simulink model "Model"  (R2021a)
settings: Solver=ode4  StartTime=0.0  StopTime=inf  FixedStep=Ts  RelTol=1e-3
PreLoadFcn:
  | filepath  = fileparts(get_param(bdroot, 'FileName'))
  | cd(filepath);
values from neighbouring files (symbols this model uses):
  A_GRotation = [0 0 0]    [Parameter_PX4.m]
  ACC_UserFault = 0    [Parameter_PX4.m]
  ACCDrift = 0.0    (= 0)    [Parameter_PX4.m]
  ACCNoise = 1.0    (= 1)    [Parameter_PX4.m]
  accnoisegain = 0    [Parameter_PX4.m]
  ACCScale = 1.0    (= 1)    [Parameter_PX4.m]
  BaroNoise = 1.0    (= 1)    [Parameter_PX4.m]
  GyroDrift = 0.0    (= 0)    [Parameter_PX4.m]
  GyroNoise = 1.0    (= 1)    [Parameter_PX4.m]
  GyroScale = 1.0    (= 1)    [Parameter_PX4.m]
  MagDrift = 0.0    (= 0)    [Parameter_PX4.m]
  MagNoise = 1.0    (= 1)    [Parameter_PX4.m]
  MagRotation = [0 0 0]    [Parameter_PX4.m]
  MagScale = 1.0    (= 1)    [Parameter_PX4.m]
  ModelInit_GroundSlope = [0,0]    [Parameter_PX4.m]
  ModelInit_RPM = 0    [Parameter_PX4.m]
  ModelParam_envAltitude = -100    [Parameter_PX4.m]
  ModelParam_GlobalNoiseGainSwitch = 0.4    [Parameter_PX4.m]
  ModelParam_GPSEphFinal = 0.3    [Parameter_PX4.m]
  ModelParam_GPSEpvFinal = 0.4    [Parameter_PX4.m]
  ModelParam_GPSFix3DFix = 3    [Parameter_PX4.m]
  ModelParam_GPSSatsVisible = 10    [Parameter_PX4.m]
  ModelParam_motorCr = 842.1    [Parameter_PX4.m]
  ModelParam_motorJm = 0.0001287    [Parameter_PX4.m]
  ModelParam_motorMinThr = 0.05    [Parameter_PX4.m]
  ModelParam_motorT = 0.0214    [Parameter_PX4.m]
  ModelParam_motorWb = 22.83    [Parameter_PX4.m]
  ModelParam_noiseBaroCoupleWithSpeed = 0    [Parameter_PX4.m]
  ModelParam_noiseUpperWindBodyRatio = 0    [Parameter_PX4.m]
  ModelParam_rotorCm = 2.783e-07    [Parameter_PX4.m]
  ModelParam_rotorCt = 1.681e-05    [Parameter_PX4.m]
  ModelParam_uavCCm = [0.0035 0.0039 0.0034]    [Parameter_PX4.m]
  ModelParam_uavCd = 0.055    [Parameter_PX4.m]
  ModelParam_uavDearo = 0.12    [Parameter_PX4.m]
  ModelParam_uavMass = 1.515    [Parameter_PX4.m]
  ModelParam_uavR = 0.225    [Parameter_PX4.m]
  ModelParam_uavType = int8(3)    [Parameter_PX4.m]
  MyNoiseGain = [2.5;3;4].*3    [Parameter_PX4.m]
  PWMNoiseGain = [10;15;3]    [Parameter_PX4.m]
  TemperatureConstant = 25.0    (= 25)    [Parameter_PX4.m]
  Ts = 1/2000    (= 0.0005)    [Parameter_PX4.m]
  TypeMotorAngMatrix = [     [pi/3 pi -pi/3 0 0 0 0 0];     [pi/3 pi -pi/3 0 0 0 0 0];     [pi/4 pi/4+pi pi/4+3*pi/2 pi/4+pi/2 0 0 0 0];     [pi/2 3*pi/2 0 pi 0 0 0 0];     [pi/2 3/2*pi 3/2*pi+pi/3 pi/2+pi/3 pi/2-pi/3 3/2*pi-pi/3 0 0];     [0 pi pi+pi/3 pi/3 -pi/3 pi-pi/3 0 0];     [pi/3 pi/3 pi pi -pi/3 -pi/3 0 0];     [pi/8 pi+pi/8 pi/8+pi/4 pi-pi/8 -pi/8 3/2*pi-pi/8 3/2*pi+pi/8 pi/2+pi/8];     [0 pi pi/4 3/4*pi -pi/4 ...(+86 chars)    [Parameter_PX4.m]
  TypeMotorDirMatrix = [     [-1 -1 -1 0 0 0 0 0];     [1 1 1 0 0 0 0 0];     [-1 -1 1 1 0 0 0 0];     [-1 -1 1 1 0 0 0 0];     [1 -1 1 -1 -1 1 0 0];     [1 -1 1 -1 -1 1 0 0];     [1 -1 1 -1 1 -1 0 0];     [1 1 -1 -1 -1 -1 1 1];     [1 1 -1 -1 -1 -1 1 1];     [-1 1 -1 1 -1 1 -1 1]; ]'    [Parameter_PX4.m]
  TypeMotorNonVector = int8([3;3;4;4;6;6;6;8;8;8])    [Parameter_PX4.m]
undefined symbols (not defined in the file or in its folder): Earth, ModelParam_GPSEpvInitial, ModelParam_GPSEpvTimeConstant, ModelParam_noiseGPSSampTime, ModelParam_noisePowerIMU, ModelParam_noisePowerOffGainAccel, ModelParam_noisePowerOffGainAccelZ, ModelParam_noisePowerOffGainGyro, ModelParam_noisePowerOffGainGyroZ, ModelParam_noisePowerOffGainMag, ModelParam_noisePowerOffGainMagZ, ModelParam_noisePowerOnGainAccel, ModelParam_noisePowerOnGainAccelZ, ModelParam_noisePowerOnGainGyro, ModelParam_noisePowerOnGainGyroZ, ModelParam_noisePowerOnGainMag, ModelParam_noisePowerOnGainMagZ, ModelParam_noiseUpperGPS, ModelParam_timeSamp, Newton, Raphson, WGS84
libraries: simulink x11, sharedtransform x7, aerolibutil x4, aerolibtransform2 x4, aerolibasang x3, simulink_extras x2, etargetslib x2, aerolibatmos2 x2, shared6dof x1, aerolibconvert2 x1, aerolibobsolete x1, aerolibnav x1
(part 1 of 3)
settings Model: SimulationMode=accelerator  ParamWorkspaceSource=ReferencedWorkspace  Creator=Jinrui  LastModifiedBy=fangr
settings SolverCC: AlgebraicLoopSolver=TrustRegion  PositivePriorityOrder=on  AutoInsertRateTranBlk=on
settings DataIOCC: ReturnWorkspaceOutputs=off
settings OptimizationCC: BlockReduction=off  EnhancedBackFolding=on  PassReuseOutputArgsAs=Individual arguments  ZeroExternalMemoryAtStartup=off  ZeroInternalMemoryAtStartup=off  OptimizeBlockOrder=speed  DifferentSizesBufferReuse=on  OptimizationCustomize=off  EfficientTunableParamExpr=on
settings DebuggingCC: ParameterTunabilityLossMsg=error  SFMachineParentedDataDiag=warning  ArithmeticOperatorsInVariantConditions=warning
settings HardwareCC: ProdBitPerPointer=32  ProdBitPerSizeT=32  ProdBitPerPtrDiffT=32  ProdLargestAtomicInteger=Long  ProdLargestAtomicFloat=Double  ProdWordSize=32  ProdHWDeviceType=ARM Compatible->ARM Cortex-A
settings SFSimCC: SimUseLocalCustomCode=off  MATLABDynamicMemAlloc=off  CustomCodeUndefinedFunction=UseInterfaceOnly
settings RTWCC: SystemTargetFile=ert.tlc  GenCodeOnly=on  PackageGeneratedCodeAndArtifacts=on  PackageName=Model  TemplateMakefile=ert_default_tmf  GenerateReport=on  RTWUseLocalCustomCode=off  Toolchain=Linaro Toolchain v4.8  BuildConfiguration=Faster Runs  DLArmComputeVersion=20.02.1
settings CodeAppCC: IgnoreCustomStorageClasses=off  OperatorAnnotations=on  SimulinkDataObjDesc=on  SFDataObjDesc=on  SimulinkBlockComments=off
settings ERTTargetCC: TargetLangStandard=C99 (ISO)  GenerateSampleERTMain=on  SupportComplex=off  SupportContinuousTime=on  SupportVariableSizeSignals=on  RootIOFormat=Structure reference  ERTCustomFileTemplate=example_file_process.tlc  ERTFilePackagingFormat=Compact
settings SimscapeCC: SimscapeNormalizeSystem=off
settings ConfigComp: DVTestSuiteOptimization=Auto  DVDetectOutOfBounds=on  DVModelReferenceHarness=on  DVHarnessSource=Signal Editor

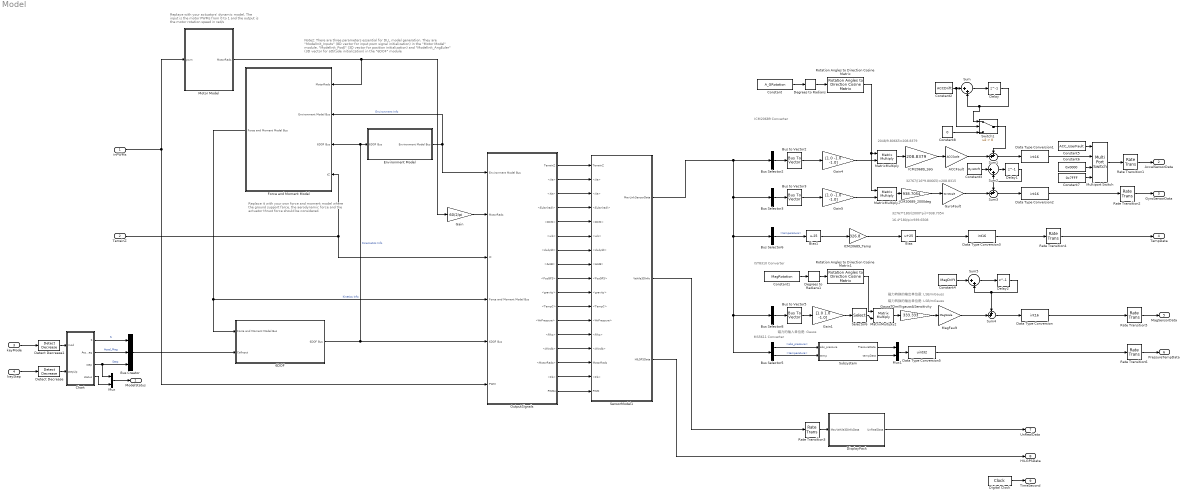
== system Model ==
  note: Replace it with your own force and moment model
      | where the ground support farce, the aerodynamic force
      | and the actuator thrust force should be considered.
  note: Replace with your actuators' dynamic model,
      | The input is the motor PWMs from 0 to 1
      | and the output is the motor rotation speed in rad/s
  note: Note2: There are three parameters essential for DLL model generation. They are "ModelInit_Inputs" (8D vector for input pwm signal initialization) in the "Motor Model" module, "ModelInit_PosE" (3D vector for position initialization) and "ModelInit_AngEuler" (3D vector for attitude initialization) in the "6DOF" module
  note: ICM20689 Converter
  note: 32767/(16*9.80665)=208.8315
  note: 2048/9.80665=208.8379
  note: 32767*180/(2000*pi)=938.7054
  note: IST8310 Converter
  note: 磁力转换的输出单位是: LSB/mGauss
  note: 磁力的输入单位是: Gauss
  note: MS5611 Converter
  note: 16.4*180/pi=939.6508
  note: 磁力转换的输出单位是: LSB/mGauss
  inPWMs : Inport  PortDimensions=8
  TerrainZ : Inport  Port=2  SampleTime=1
  keyMode : Inport  Port=3
  keyStep : Inport  Port=4
  6DOF : Subsystem
  ACCFault : Gain  Gain=ACCScale  OutDataTypeStr=double  RndMeth=Nearest
  Bias : Bias  Bias=25
  Bias1 : Bias  Bias=-25
  Bus Creator : BusCreator  Inputs=3
  Bus Selector2 : BusSelector  OutputSignals=xacc,yacc,zacc  OutputAsBus=on
  Bus Selector3 : BusSelector  OutputSignals=xgyro,ygyro,zgyro  OutputAsBus=on
  Bus Selector5 : BusSelector  OutputSignals=abs_pressure,temperature
  Bus Selector6 : BusSelector  OutputSignals=temperature
  Bus Selector8 : BusSelector  OutputSignals=xmag,ymag,zmag  OutputAsBus=on
  Bus to Vector2 : BusToVector
  Bus to Vector3 : BusToVector
  Bus to Vector5 : BusToVector
  Chart : Stateflow chart  TreatAsAtomicUnit=on
  Constant : Constant  Value=A_GRotation
  Constant1 : Constant  Value=MagRotation
  Constant2 : Constant  Value=ACCDrift
  Constant3 : Constant  Value=GyroDrift
  Constant4 : Constant  Value=MagDrift
  Constant5 : Constant  Value=ACC_UserFault
  Constant6 : Constant  Value=0x0000  OutDataTypeStr=int16
  Constant7 : Constant  Value=0x7FFF  OutDataTypeStr=int16
  Constant8 : Constant  Value=0
  Data Type Conversion : DataTypeConversion  OutDataTypeStr=int16  RndMeth=Nearest
  Data Type Conversion1 : DataTypeConversion  OutDataTypeStr=int16  RndMeth=Nearest  SaturateOnIntegerOverflow=on
  Data Type Conversion2 : DataTypeConversion  OutDataTypeStr=int16  RndMeth=Nearest  SaturateOnIntegerOverflow=on
  Data Type Conversion3 : DataTypeConversion  OutDataTypeStr=int16  RndMeth=Nearest
  Data Type Conversion5 : DataTypeConversion  OutDataTypeStr=uint32  RndMeth=Nearest
  Degrees to Radians : simulink_extras/Transformations/Degrees to Radians
  Degrees to Radians1 : simulink_extras/Transformations/Degrees to Radians
  Delay : Delay  DelayLength=1
  Delay1 : Delay  DelayLength=1
  Delay2 : Delay  DelayLength=1
  Detect Decrease : simulink/Logic and Bit Operations/Detect Decrease  vinit=0.0  OutDataTypeStr=boolean
  Detect Decrease1 : simulink/Logic and Bit Operations/Detect Decrease  vinit=0.0  OutDataTypeStr=boolean
  Digital Clock : DigitalClock  SampleTime=Ts
  DisplayPack : Subsystem  TreatAsAtomicUnit=on  SystemSampleTime=Ts
  Environment Model : Subsystem
  Force and Moment Model : Subsystem
  Gain : Gain  Gain=60/2/pi
  Gain1 : Gain  Gain=[1.0 1.0 -1.0]  RndMeth=Nearest
  Gain4 : Gain  Gain=[1.0 -1.0 -1.0]  RndMeth=Nearest
  Gain5 : Gain  Gain=[1.0 -1.0 -1.0]  RndMeth=Nearest
  GaussTOmilligauss&Sensitivity : Gain  Gain=333.333  OutDataTypeStr=double  RndMeth=Nearest
  GyroFault : Gain  Gain=GyroScale  OutDataTypeStr=double  RndMeth=Nearest
  ICM20689_16G : Gain  Gain=208.8379  OutDataTypeStr=double  RndMeth=Nearest
  ICM20689_2000deg : Gain  Gain=938.7054  OutDataTypeStr=double  RndMeth=Nearest
  ICM20689_Temp : Gain  Gain=326.8  OutDataTypeStr=double
  MagFault : Gain  Gain=MagScale  OutDataTypeStr=double  RndMeth=Nearest
  MatrixMultiply : Product  Multiplication=Matrix(*)
  MatrixMultiply1 : Product  Multiplication=Matrix(*)
  MatrixMultiply2 : Product  Multiplication=Matrix(*)
  Motor Model : Subsystem
  Multiport Switch : MultiPortSwitch  DataPortOrder=Specify indices  DataPortIndices={0,1,2}  DiagnosticForDefault=None
  Mux : Mux  Inputs=2
  Mux1 : Mux  Inputs=2
  OutputSignals : Subsystem
  Rate Transition1 : RateTransition  OutPortSampleTime=Ts*2
  Rate Transition2 : RateTransition  OutPortSampleTime=Ts
  Rate Transition3 : RateTransition  OutPortSampleTime=0.01
  Rate Transition4 : RateTransition  OutPortSampleTime=Ts
  Rate Transition5 : RateTransition  OutPortSampleTime=Ts
  Rate Transition6 : RateTransition  OutPortSampleTime=Ts*2
  Rotation Angles to Direction Cosine Matrix : sharedtransform/Rotation Angles to Direction Cosine Matrix  rotationOrder=ZYX  aMode=aMode
      settings: SourceProductBaseCode=AE,PW,DR,MT,VE
  Rotation Angles to Direction Cosine Matrix1 : sharedtransform/Rotation Angles to Direction Cosine Matrix  rotationOrder=ZYX  aMode=aMode
      settings: SourceProductBaseCode=AE,PW,DR,MT,VE
  Selector6 : Selector  InputPortWidth=3  IndexOptions=Index vector (dialog)  Indices=[2 1 3]  OutputSizes=1
  SensorModel1 : Subsystem
  Subsystem : Subsystem
  Sum : Sum  Inputs=|++
  Sum1 : Sum  Inputs=++|
  Sum2 : Sum  Inputs=|++
  Sum3 : Sum  Inputs=++|
  Sum4 : Sum  Inputs=++|
  Sum5 : Sum  Inputs=|++
  Switch1 : Switch  Criteria=u2 > Threshold
  ModelStatus : Outport  PortDimensions=2
  AccelSensorData : Outport  Port=2  OutDataTypeStr=int16
  GyroSensorData : Outport  Port=3
  TempData : Outport  Port=4
  MagSensorData : Outport  Port=5
  PressureTempData : Outport  Port=6
  UnRealData : Outport  Port=7
  HILGPSData : Outport  Port=8
  TimeSecond : Outport  Port=9
  wires:
  inPWMs/1 -> Motor Model/1(pwm), OutputSignals/6(PWM)
  OutputSignals/7(<dwb/dt>) -> SensorModel1/7(<dwb/dt>)
  OutputSignals/13(<Rho>) -> SensorModel1/13(<Rho>)
  OutputSignals/6(<wb>) -> SensorModel1/6(<wb>)
  OutputSignals/12(<AirPressure>) -> SensorModel1/12(<AirPressure>)
  OutputSignals/9(<PosGPS>) -> SensorModel1/9(<PosGPS>)
  Environment Model/1(Environment Model Bus) -> Force and Moment Model/2(Environment Model Bus), OutputSignals/1(Environment Model Bus)  "Environment Info"
  OutputSignals/17(PWMs) -> SensorModel1/17(PWM)
  OutputSignals/11(<TempC>) -> SensorModel1/11(<TempC>)
  OutputSignals/10(<gravity>) -> SensorModel1/10(<gravity>)
  TerrainZ/1 -> Force and Moment Model/4("tZ "), OutputSignals/3(zt)
  OutputSignals/8(<AccB>) -> SensorModel1/8(<AccB>)
  Chart/3(step) -> Mux/1, Bus Creator/3  "Step"
  Chart/2(Accel_Mag) -> Bus Creator/2  "Accel_Mag"
  Detect Decrease1/1 -> Chart/1(mod)
  Force and Moment Model/1(Force and Moment Model Bus) -> OutputSignals/4(Force and Moment Model Bus), 6DOF/1(Force and Moment Model Bus)  "Kinetics Info"
  OutputSignals/2(<Ve>) -> SensorModel1/2(<Ve>)
  OutputSignals/1(TerrainZ) -> SensorModel1/1(TerrainZ)
  OutputSignals/4(<Eular(rad)>) -> SensorModel1/4(<Eular(rad)>)
  6DOF/1(6DOF Bus) -> Force and Moment Model/3(6DOF Bus), Environment Model/1(6DOF Bus), OutputSignals/5(6DOF Bus)  "Kinematics Info"
  OutputSignals/3(<Xe>) -> SensorModel1/3(<Xe>)
  Motor Model/1(MotorRads) -> Force and Moment Model/1(MotorRads), Gain/1
  OutputSignals/15(<MotorRads>) -> SensorModel1/15(MotorRads)
  OutputSignals/16(<Fb>) -> SensorModel1/16(<Fb>)
  OutputSignals/14(<Windb>) -> SensorModel1/14(<Windb>)
  Detect Decrease/1 -> Chart/2(stepUp)
  keyMode/1 -> Detect Decrease1/1
  Chart/4(status) -> Mux/2
  Chart/1(S) -> Bus Creator/1  "S"
  OutputSignals/5(<DCM>) -> SensorModel1/5(<DCM>)
  keyStep/1 -> Detect Decrease/1
  Bus Creator/1 -> 6DOF/2(CalInput)
  Mux/1 -> ModelStatus/1
  Gain/1 -> OutputSignals/2(MotorRads)
  Sum2/1 -> Delay1/1
  ACCFault/1 -> Sum1/2
  Constant3/1 -> Sum2/1
  Delay1/1 -> Sum3/1, Sum2/2
  ICM20689_Temp/1 -> Bias/1
  Delay/1 -> Switch1/1, Sum/2
  Degrees to Radians1/1 -> Rotation Angles to Direction Cosine Matrix1/1
  Bus Selector5/1 -> Subsystem/1(abs_pressure)  "<abs_pressure>"
  Rotation Angles to Direction Cosine Matrix1/1 -> MatrixMultiply2/1
  MagFault/1 -> Sum4/2
  GyroFault/1 -> Sum3/2
  Sum/1 -> Delay/1
  SensorModel1/2(Vehile3DInfo) -> Rate Transition3/1
  Constant1/1 -> Degrees to Radians1/1
  MatrixMultiply1/1 -> ICM20689_2000deg/1
  Subsystem/2(tempData) -> Mux1/2
  Constant4/1 -> Sum5/1
  Rate Transition3/1 -> DisplayPack/1(MavVehile3DInfoData)
  Sum5/1 -> Delay2/1
  Sum3/1 -> Data Type Conversion2/1
  ICM20689_16G/1 -> ACCFault/1
  ICM20689_2000deg/1 -> GyroFault/1
  Bus Selector8/1 -> Bus to Vector5/1
  SensorModel1/1(MavLinkSensorData) -> Bus Selector3/1, Bus Selector6/1, Bus Selector8/1, Bus Selector5/1, Bus Selector2/1
  DisplayPack/1(UnRealData) -> UnRealData/1
  Mux1/1 -> Data Type Conversion5/1
  Sum4/1 -> Data Type Conversion/1
  Delay2/1 -> Sum4/1, Sum5/2
  Selector6/1 -> MatrixMultiply2/2
  Bus Selector6/1 -> Bias1/1  "<temperature>"
  Bias/1 -> Data Type Conversion3/1
  Sum1/1 -> Data Type Conversion1/1
  Bus Selector3/1 -> Bus to Vector3/1
  Degrees to Radians/1 -> Rotation Angles to Direction Cosine Matrix/1
  Constant2/1 -> Switch1/2, Sum/1
  Bus Selector2/1 -> Bus to Vector2/1
  Bus to Vector5/1 -> Gain1/1
  Bias1/1 -> ICM20689_Temp/1
  Bus to Vector3/1 -> Gain5/1
  SensorModel1/3(HILGPSData) -> HILGPSData/1
  Gain1/1 -> Selector6/1
  Constant/1 -> Degrees to Radians/1
  Subsystem/1(PressureData) -> Mux1/1
  Bus Selector5/2 -> Subsystem/2(temp)  "<temperature>"
  MatrixMultiply2/1 -> GaussTOmilligauss&Sensitivity/1
  Gain4/1 -> MatrixMultiply/2
  GaussTOmilligauss&Sensitivity/1 -> MagFault/1
  MatrixMultiply/1 -> ICM20689_16G/1
  Bus to Vector2/1 -> Gain4/1
  Constant5/1 -> Multiport Switch/1
  Data Type Conversion1/1 -> Multiport Switch/2
  Constant6/1 -> Multiport Switch/3
  Constant7/1 -> Multiport Switch/4
  Gain5/1 -> MatrixMultiply1/2
  Digital Clock/1 -> TimeSecond/1
  Multiport Switch/1 -> Rate Transition1/1
  Rate Transition1/1 -> AccelSensorData/1
  Rate Transition2/1 -> GyroSensorData/1
  Data Type Conversion2/1 -> Rate Transition2/1
  Rate Transition4/1 -> TempData/1
  Data Type Conversion3/1 -> Rate Transition4/1
  Data Type Conversion/1 -> Rate Transition5/1
  Rate Transition5/1 -> MagSensorData/1
  Data Type Conversion5/1 -> Rate Transition6/1
  Rate Transition6/1 -> PressureTempData/1
  Rotation Angles to Direction Cosine Matrix/1 -> MatrixMultiply/1, MatrixMultiply1/1
  Constant8/1 -> Switch1/3
  Switch1/1 -> Sum1/1

== system Model/6DOF ==
  Force and Moment Model Bus : Inport
  CalInput : Inport  Port=2
  Bus Creator : BusCreator  Inputs=8
  Bus Selector : BusSelector  OutputSignals=Step,Accel_Mag,S
  Bus Selector1 : BusSelector  OutputSignals=Fb,Mb
  CaliModel : Subsystem
  Custom Variable Mass 6DOF (Quaternion) : shared6dof/6DOF (Euler Angles)  units=Metric (MKS)  mtype=Fixed  rep=Quaternion  xme_0=ModelInit_PosE  Vm_0=ModelInit_VelB  eul_0=ModelInit_AngEuler  pm_0=ModelInit_RateB  mass_0=ModelParam_uavMass  mass_e=0.5  mass_f=2.0  inertia=ModelParam_uavJ  inertia_e=eye(3)  inertia_f=2*eye(3)  k_quat=1.0  vre_flag=off  abi_flag=off  aMode=aMode  xme_statename=''  Vm_statename=''  eul_statename=''  quat_statename=''  pm_statename=''  mass_statename=''
      settings: SourceProductBaseCode=AE,PW,DR,MT,VE
  Demux2 : Demux  Outputs=3
  Mux : Mux  Inputs=3
  Switch : Switch  Criteria=u2 > Threshold
  Switch1 : Switch  Criteria=u2 > Threshold
  Wrap To Zero : simulink/Discontinuities/Wrap To Zero  Threshold=0
      settings: SourceProductBaseCode=SL
  6DOF Bus : Outport  VectorParamsAs1DForOutWhenUnconnected=off
  wires:
  Bus Selector1/1 -> Switch/1  "<Fb>"
  Custom Variable Mass 6DOF (Quaternion)/8 -> Bus Creator/8  "AccB"
  Custom Variable Mass 6DOF (Quaternion)/5 -> Bus Creator/5  "Vb"
  Custom Variable Mass 6DOF (Quaternion)/6 -> Bus Creator/6, CaliModel/3(wb)  "wb"
  Custom Variable Mass 6DOF (Quaternion)/1 -> Bus Creator/1  "Ve"
  Custom Variable Mass 6DOF (Quaternion)/4 -> CaliModel/4(DCM_be), Bus Creator/4  "DCM"
  Custom Variable Mass 6DOF (Quaternion)/3 -> Bus Creator/3  "Eular(rad)"
  Custom Variable Mass 6DOF (Quaternion)/7 -> Bus Creator/7  "dwb/dt"
  Bus Selector1/2 -> Switch1/1  "<Mb>"
  Force and Moment Model Bus/1 -> Bus Selector1/1
  Bus Creator/1 -> 6DOF Bus/1
  Bus Selector/3 -> Switch/2, Switch1/2  "<S>"
  Bus Selector/2 -> CaliModel/2(Accel_Mag)  "<Accel_Mag>"
  Bus Selector/1 -> CaliModel/1(step)  "<Step>"
  CalInput/1 -> Bus Selector/1
  Switch/1 -> Custom Variable Mass 6DOF (Quaternion)/1
  Switch1/1 -> Custom Variable Mass 6DOF (Quaternion)/2
  CaliModel/1(Fb) -> Switch/3
  CaliModel/2(Mb) -> Switch1/3
  Demux2/1 -> Mux/1
  Demux2/2 -> Mux/2
  Demux2/3 -> Wrap To Zero/1
  Wrap To Zero/1 -> Mux/3
  Custom Variable Mass 6DOF (Quaternion)/2 -> Demux2/1  "Xe"
  Mux/1 -> Bus Creator/2  "Xe"

== system Model/DisplayPack ==
  MavVehile3DInfoData : Inport
  Bus Selector : BusSelector  OutputSignals=copterID,vehicleType,runnedTime,VelE,PosE,AngEuler,AngQuatern,MotorRPMS,AccB,RateB,PosGPS
  UnRealDataPackege : Subsystem  TreatAsAtomicUnit=on
  UnRealData : Outport
  wires:
  UnRealDataPackege/1(toUnReal) -> UnRealData/1
  MavVehile3DInfoData/1 -> Bus Selector/1
  Bus Selector/1 -> UnRealDataPackege/1(copterID)  "<copterID>"
  Bus Selector/2 -> UnRealDataPackege/2(vehicleType)  "<vehicleType>"
  Bus Selector/3 -> UnRealDataPackege/3(runnedTime)  "<runnedTime>"
  Bus Selector/4 -> UnRealDataPackege/4("VelE ")  "<VelE>"
  Bus Selector/5 -> UnRealDataPackege/5(PosE)  "<PosE>"
  Bus Selector/6 -> UnRealDataPackege/6(AngEuler)  "<AngEuler>"
  Bus Selector/7 -> UnRealDataPackege/7(AngQuatern)  "<AngQuatern>"
  Bus Selector/8 -> UnRealDataPackege/8(MotorRPMS)  "<MotorRPMS>"
  Bus Selector/9 -> UnRealDataPackege/9(AccB)  "<AccB>"
  Bus Selector/10 -> UnRealDataPackege/10(RateB)  "<RateB>"
  Bus Selector/11 -> UnRealDataPackege/11(PosGPS)  "<PosGPS>"

== system Model/Environment Model ==
  6DOF Bus : Inport
  Bus Creator : BusCreator  Inputs=6
  Bus Selector : BusSelector  OutputSignals=Xe,Vb
  Constant_[1 1 1] : Constant  Value=[1,1,1]  VectorParams1D=off
  Flat Earth to LLA : aerolibtransform2/Flat Earth to LLA  units=Metric (MKS)  ptype=Earth (WGS84)  F=1/298.257223563  R=6378137  refPosPort=off  LL0=ModelParam_GPSLatLong  psi=0
  ISA Atmosphere Model : aerolibatmos2/ISA Atmosphere Model  custom=off  g=9.80665  gamma=1.4  R=287.0531  L=0.0065  h_trop=11000  h_strat=20000  rho0=1.225  P0=101325  T0=288.15  h0=0
  ModelParam.envAltitude : Constant  Value=ModelParam_envAltitude
  ModelParam.noiseUpperWindBodyRatio : Gain  Gain=ModelParam_noiseUpperWindBodyRatio
  ModelParam.noiseUpperWindBodyRatioSwitch : Gain  Gain=ModelParam_GlobalNoiseGainSwitch
  Mux : Mux  Inputs=2
  Product1 : Product
  Reshape : Reshape
  Saturation : Saturate  UpperLimit=100000  LowerLimit=0
  Sum1 : Sum  Inputs=|++
  Temperature Conversion : aerolibconvert2/Temperature Conversion  IU=K  OU=C
      settings: SourceProductBaseCode=AE
  TemperatureConstant : Constant  Value=TemperatureConstant
  Terminator2 : Terminator
  Terminator3 : Terminator
  Uniform Random Number : UniformRandomNumber  Minimum=[-1,-1,-0.5]  Maximum=[1,1,0.5]  Seed=[564565,6846798,46545]  SampleTime=Ts
  "WGS84 Gravity Model " : aerolibobsolete/WGS84 Gravity Model   model=WGS84 Taylor Series  units=Metric (MKS)  no_atmos=on  precessing=on  jd_loc=off  month=October  day=10  year=2004  no_centrifugal=on  action=Warning
      settings: SourceProductBaseCode=AE
  Environment Model Bus : Outport  VectorParamsAs1DForOutWhenUnconnected=off
  wires:
  ModelParam.envAltitude/1 -> Flat Earth to LLA/2
  Bus Creator/1 -> Environment Model Bus/1
  Bus Selector/1 -> Flat Earth to LLA/1  "<Xe>"
  Constant_[1 1 1]/1 -> Sum1/1
  ModelParam.noiseUpperWindBodyRatioSwitch/1 -> Sum1/2
  ModelParam.noiseUpperWindBodyRatio/1 -> ModelParam.noiseUpperWindBodyRatioSwitch/1
  6DOF Bus/1 -> Bus Selector/1
  ISA Atmosphere Model/3 -> Bus Creator/4  "AirPressure"
  "WGS84 Gravity Model "/1 -> Reshape/1
  TemperatureConstant/1 -> Bus Creator/3  "TempC"
  ISA Atmosphere Model/4 -> Bus Creator/5  "Rho"
  Uniform Random Number/1 -> ModelParam.noiseUpperWindBodyRatio/1
  Reshape/1 -> Bus Creator/2  "gravity"
  Product1/1 -> Bus Creator/6  "Windb"
  Flat Earth to LLA/1 -> Mux/1
  Temperature Conversion/1 -> Terminator2/1
  Mux/1 -> Bus Creator/1, "WGS84 Gravity Model "/1  "PosGPS"
  ISA Atmosphere Model/2 -> Terminator3/1
  ISA Atmosphere Model/1 -> Temperature Conversion/1
  Bus Selector/2 -> Product1/2  "<Vb>"
  Flat Earth to LLA/2 -> Mux/2, Saturation/1
  Sum1/1 -> Product1/1
  Saturation/1 -> ISA Atmosphere Model/1

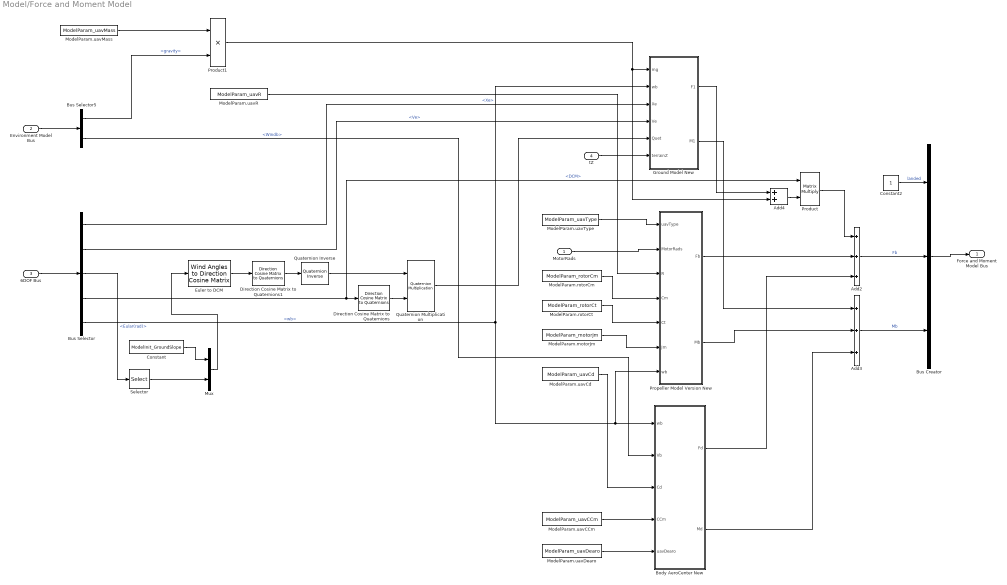
== system Model/Force and Moment Model ==
  MotorRads : Inport
  Environment Model Bus : Inport  Port=2
  6DOF Bus : Inport  Port=3
  "tZ " : Inport  Port=4
  Add2 : Sum  Inputs=+++
  Add3 : Sum  Inputs=+++
  Add4 : Sum
  Body AeroCenter New : Subsystem
  Bus Creator : BusCreator  Inputs=3
  Bus Selector : BusSelector  OutputSignals=Xe,Ve,Eular(rad),DCM,wb
  Bus Selector5 : BusSelector  OutputSignals=gravity,Windb
  Constant : Constant  Value=ModelInit_GroundSlope
  Constant2 : Constant
  Direction Cosine Matrix to Quaternions : sharedtransform/Direction Cosine Matrix  to Quaternions  aMode=aMode  action=None  tolerance=eps(2)
      settings: SourceProductBaseCode=AE
  Direction Cosine Matrix to Quaternions1 : sharedtransform/Direction Cosine Matrix  to Quaternions  aMode=aMode  action=None  tolerance=eps(2)
      settings: SourceProductBaseCode=AE
  Euler to DCM : aerolibtransform2/Wind Angles to  Direction Cosine Matrix
      settings: SourceProductBaseCode=AE
  Ground Model New : Subsystem
  ModelParam.motorJm : Constant  Value=ModelParam_motorJm
  ModelParam.rotorCm : Constant  Value=ModelParam_rotorCm
  ModelParam.rotorCt : Constant  Value=ModelParam_rotorCt
  ModelParam.uavCCm : Constant  Value=ModelParam_uavCCm
  ModelParam.uavCd : Constant  Value=ModelParam_uavCd
  ModelParam.uavDearo : Constant  Value=ModelParam_uavDearo
  ModelParam.uavMass : Constant  Value=ModelParam_uavMass
  ModelParam.uavR : Constant  Value=ModelParam_uavR
  ModelParam.uavType : Constant  Value=ModelParam_uavType
  Mux : Mux  Inputs=2
  Product : Product  Multiplication=Matrix(*)
  Product1 : Product
  Propeller Model Version New : Subsystem
  Quaternion Inverse : aerolibutil/Quaternion Inverse
  Quaternion Multiplication : aerolibutil/Quaternion Multiplication
  Selector : Selector  InputPortWidth=3  IndexOptions=Index vector (dialog)  Indices=[3]  OutputSizes=1
  Force and Moment Model Bus : Outport  VectorParamsAs1DForOutWhenUnconnected=off
  wires:
  Body AeroCenter New/2(Md) -> Add3/3
  Body AeroCenter New/1(Fd) -> Add2/3
  Constant2/1 -> Bus Creator/1  "landed"
  "tZ "/1 -> Ground Model New/6(terrainZ)
  Add3/1 -> Bus Creator/3  "Mb"
  Add2/1 -> Bus Creator/2  "Fb"
  Quaternion Multiplication/1 -> Ground Model New/5(Quet)
  Quaternion Inverse/1 -> Quaternion Multiplication/1
  Direction Cosine Matrix to Quaternions1/1 -> Quaternion Inverse/1
  Euler to DCM/1 -> Direction Cosine Matrix to Quaternions1/1
  Mux/1 -> Euler to DCM/1
  Direction Cosine Matrix to Quaternions/1 -> Quaternion Multiplication/2
  Product/1 -> Add2/1
  Ground Model New/1(F1) -> Add4/1
  Add4/1 -> Product/2
  Product1/1 -> Ground Model New/1(mg), Add4/2
  Ground Model New/2(M1) -> Add3/1
  Bus Selector/4 -> Direction Cosine Matrix to Quaternions/1, Product/1  "<DCM>"
  ModelParam.uavCd/1 -> Body AeroCenter New/3(Cd)
  Bus Selector/5 -> Ground Model New/2(wb), Body AeroCenter New/1(wb), Propeller Model Version New/7(wb)  "<wb>"
  ModelParam.uavCCm/1 -> Body AeroCenter New/4(CCm)
  Bus Creator/1 -> Force and Moment Model Bus/1
  6DOF Bus/1 -> Bus Selector/1
  Bus Selector/2 -> Ground Model New/4(Ve)  "<Ve>"
  Bus Selector/1 -> Ground Model New/3(Xe)  "<Xe>"
  Bus Selector/3 -> Selector/1  "<Eular(rad)>"
  ModelParam.uavMass/1 -> Product1/1
  Bus Selector5/1 -> Product1/2  "<gravity>"
  Environment Model Bus/1 -> Bus Selector5/1
  Bus Selector5/2 -> Body AeroCenter New/2(Vb)  "<Windb>"
  ModelParam.uavDearo/1 -> Body AeroCenter New/5(uavDearo)
  ModelParam.uavR/1 -> Propeller Model Version New/3(R)
  ModelParam.uavType/1 -> Propeller Model Version New/1(uavType)
  MotorRads/1 -> Propeller Model Version New/2(MotorRads)
  ModelParam.motorJm/1 -> Propeller Model Version New/6(Jm)
  Propeller Model Version New/2(Mb) -> Add3/2
  Propeller Model Version New/1(Fb) -> Add2/2
  ModelParam.rotorCm/1 -> Propeller Model Version New/4(Cm)
  ModelParam.rotorCt/1 -> Propeller Model Version New/5(Ct)
  Selector/1 -> Mux/2
  Constant/1 -> Mux/1

== system Model/Motor Model ==
  pwm : Inport
  Constant : Constant  Value=ModelInit_RPM
  Demux : Demux  Outputs=8
  ModelParam.motorCr : Constant  Value=ModelParam_motorCr
  ModelParam.motorT : Constant  Value=ModelParam_motorT
  ModelParam.motorWb : Constant  Value=ModelParam_motorWb
  MotorNonlinearDynamic1 : Subsystem  TreatAsAtomicUnit=on
  MotorNonlinearDynamic2 : Subsystem  TreatAsAtomicUnit=on
  MotorNonlinearDynamic3 : Subsystem  TreatAsAtomicUnit=on
  MotorNonlinearDynamic4 : Subsystem  TreatAsAtomicUnit=on
  MotorNonlinearDynamic5 : Subsystem  TreatAsAtomicUnit=on
  MotorNonlinearDynamic6 : Subsystem  TreatAsAtomicUnit=on
  MotorNonlinearDynamic7 : Subsystem  TreatAsAtomicUnit=on
  MotorNonlinearDynamic8 : Subsystem  TreatAsAtomicUnit=on
  Mux : Mux  Inputs=8
  MotorRads : Outport  VectorParamsAs1DForOutWhenUnconnected=off
  wires:
  Mux/1 -> MotorRads/1
  Demux/1 -> MotorNonlinearDynamic1/5(PWM)
  MotorNonlinearDynamic1/1(radW) -> Mux/1
  ModelParam.motorCr/1 -> MotorNonlinearDynamic1/2(Cr), MotorNonlinearDynamic2/2(Cr), MotorNonlinearDynamic3/2(Cr), MotorNonlinearDynamic4/2(Cr), MotorNonlinearDynamic5/2(Cr), MotorNonlinearDynamic6/2(Cr), MotorNonlinearDynamic8/2(Cr), MotorNonlinearDynamic7/2(Cr)
  ModelParam.motorWb/1 -> MotorNonlinearDynamic1/1(Wb), MotorNonlinearDynamic2/1(Wb), MotorNonlinearDynamic3/1(Wb), MotorNonlinearDynamic4/1(Wb), MotorNonlinearDynamic5/1(Wb), MotorNonlinearDynamic6/1(Wb), MotorNonlinearDynamic8/1(Wb), MotorNonlinearDynamic7/1(Wb)
  Demux/2 -> MotorNonlinearDynamic2/5(PWM)
  Demux/3 -> MotorNonlinearDynamic3/5(PWM)
  Demux/4 -> MotorNonlinearDynamic4/5(PWM)
  Demux/5 -> MotorNonlinearDynamic5/5(PWM)
  Demux/6 -> MotorNonlinearDynamic6/5(PWM)
  Demux/7 -> MotorNonlinearDynamic7/5(PWM)
  Demux/8 -> MotorNonlinearDynamic8/5(PWM)
  ModelParam.motorT/1 -> MotorNonlinearDynamic2/3(motorT), MotorNonlinearDynamic3/3(motorT), MotorNonlinearDynamic4/3(motorT), MotorNonlinearDynamic5/3(motorT), MotorNonlinearDynamic6/3(motorT), MotorNonlinearDynamic8/3(motorT), MotorNonlinearDynamic7/3(motorT), MotorNonlinearDynamic1/3(motorT)
  MotorNonlinearDynamic2/1(radW) -> Mux/2
  MotorNonlinearDynamic8/1(radW) -> Mux/8
  MotorNonlinearDynamic7/1(radW) -> Mux/7
  MotorNonlinearDynamic6/1(radW) -> Mux/6
  MotorNonlinearDynamic5/1(radW) -> Mux/5
  MotorNonlinearDynamic4/1(radW) -> Mux/4
  MotorNonlinearDynamic3/1(radW) -> Mux/3
  pwm/1 -> Demux/1
  Constant/1 -> MotorNonlinearDynamic8/4(ModelInit_RPM), MotorNonlinearDynamic7/4(ModelInit_RPM), MotorNonlinearDynamic6/4(ModelInit_RPM), MotorNonlinearDynamic5/4(ModelInit_RPM), MotorNonlinearDynamic4/4(ModelInit_RPM), MotorNonlinearDynamic3/4(ModelInit_RPM), MotorNonlinearDynamic2/4(ModelInit_RPM), MotorNonlinearDynamic1/4(ModelInit_RPM)

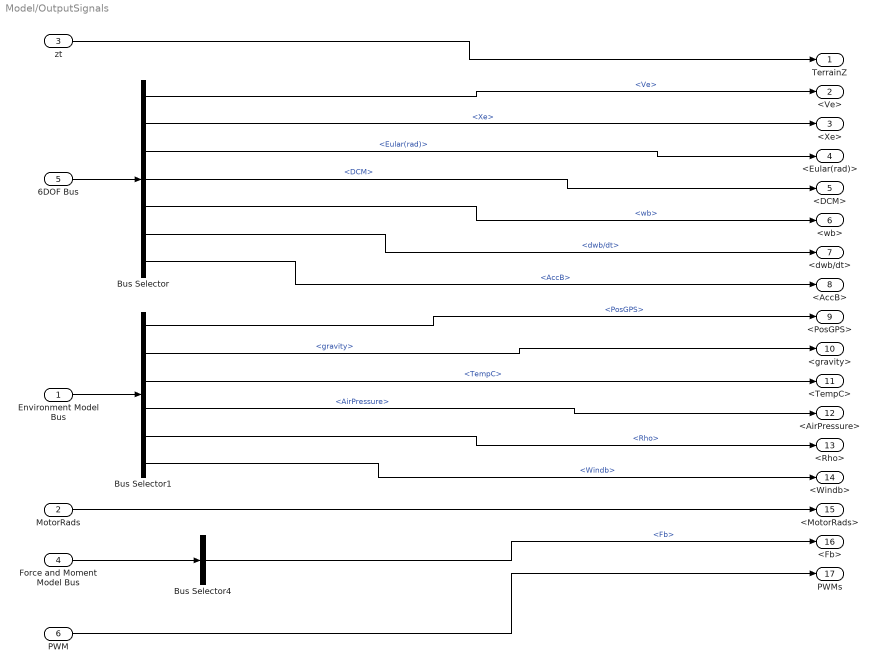
== system Model/OutputSignals ==
  Environment Model Bus : Inport
  MotorRads : Inport  Port=2
  zt : Inport  Port=3
  Force and Moment Model Bus : Inport  Port=4
  6DOF Bus : Inport  Port=5
  PWM : Inport  Port=6
  Bus Selector : BusSelector  OutputSignals=Ve,Xe,Eular(rad),DCM,wb,dwb/dt,AccB
  Bus Selector1 : BusSelector  OutputSignals=PosGPS,gravity,TempC,AirPressure,Rho,Windb
  Bus Selector4 : BusSelector  OutputSignals=Fb
  TerrainZ : Outport  VectorParamsAs1DForOutWhenUnconnected=off
  <Ve> : Outport  Port=2  VectorParamsAs1DForOutWhenUnconnected=off
  <Xe> : Outport  Port=3  VectorParamsAs1DForOutWhenUnconnected=off
  <Eular(rad)> : Outport  Port=4  VectorParamsAs1DForOutWhenUnconnected=off
  <DCM> : Outport  Port=5  VectorParamsAs1DForOutWhenUnconnected=off
  <wb> : Outport  Port=6  VectorParamsAs1DForOutWhenUnconnected=off
  <dwb/dt> : Outport  Port=7  VectorParamsAs1DForOutWhenUnconnected=off
  <AccB> : Outport  Port=8  VectorParamsAs1DForOutWhenUnconnected=off
  <PosGPS> : Outport  Port=9  VectorParamsAs1DForOutWhenUnconnected=off
  <gravity> : Outport  Port=10  VectorParamsAs1DForOutWhenUnconnected=off
  <TempC> : Outport  Port=11  VectorParamsAs1DForOutWhenUnconnected=off
  <AirPressure> : Outport  Port=12  VectorParamsAs1DForOutWhenUnconnected=off
  <Rho> : Outport  Port=13  VectorParamsAs1DForOutWhenUnconnected=off
  <Windb> : Outport  Port=14  VectorParamsAs1DForOutWhenUnconnected=off
  <MotorRads> : Outport  Port=15  VectorParamsAs1DForOutWhenUnconnected=off
  <Fb> : Outport  Port=16  VectorParamsAs1DForOutWhenUnconnected=off
  PWMs : Outport  Port=17  VectorParamsAs1DForOutWhenUnconnected=off
  wires:
  Force and Moment Model Bus/1 -> Bus Selector4/1
  MotorRads/1 -> <MotorRads>/1
  Bus Selector1/4 -> <AirPressure>/1  "<AirPressure>"
  Bus Selector/3 -> <Eular(rad)>/1  "<Eular(rad)>"
  Bus Selector1/6 -> <Windb>/1  "<Windb>"
  Bus Selector1/2 -> <gravity>/1  "<gravity>"
  PWM/1 -> PWMs/1
  Bus Selector/4 -> <DCM>/1  "<DCM>"
  Bus Selector/6 -> <dwb/dt>/1  "<dwb/dt>"
  Bus Selector1/1 -> <PosGPS>/1  "<PosGPS>"
  Bus Selector4/1 -> <Fb>/1  "<Fb>"
  Bus Selector/7 -> <AccB>/1  "<AccB>"
  Bus Selector/1 -> <Ve>/1  "<Ve>"
  Bus Selector/5 -> <wb>/1  "<wb>"
  Bus Selector/2 -> <Xe>/1  "<Xe>"
  Bus Selector1/5 -> <Rho>/1  "<Rho>"
  zt/1 -> TerrainZ/1
  Bus Selector1/3 -> <TempC>/1  "<TempC>"
  Environment Model Bus/1 -> Bus Selector1/1
  6DOF Bus/1 -> Bus Selector/1

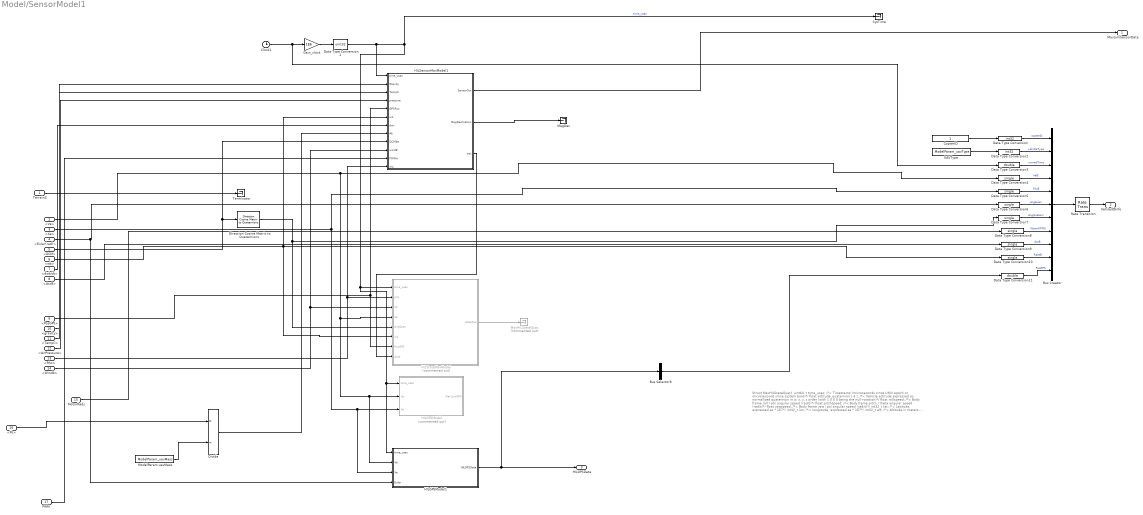
== system Model/SensorModel1 ==
  note: Struct MavHILStateQuat{
      | uint64_t time_usec; /*< Timestamp (microseconds since UNIX epoch or microseconds since system boot)*/
      | float attitude_quaternion [ 4 ]; /*< Vehicle attitude expressed as normalized quaternion in w, x, y, z order (with 1 0 0 0 being the null-rotation)*/
      | float rollspeed; /*< Body frame roll / phi angular speed (rad/s)*/
      | float pitchspeed; /*< Body frame pitch / theta angular speed (rad/s)*/
      | float yawspeed; /*< Body frame yaw / psi angular speed (rad/s)*/
      | int32_t lat; /*< Latitude, expressed as * 1E7*/
      | int32_t lon; /*< Longitude, expressed as * 1E7*/
      | int32_t alt; /*< Altitude in meters, expressed as * 1000 (millimeters)*/
      | int16_t vx; /*< Ground X Speed (Latitude), expressed as cm/s*/
      | int16_t vy; /*< Ground Y Speed (Longitude), expressed as cm/s*/
      | int16_t vz; /*< Ground Z Speed (Altitude), expressed as cm/s*/
      | uint16_t ind_airspeed; /*< Indicated airspeed, expressed as cm/s*/
      | uint16_t true_airspeed; /*< True airspeed, expressed as cm/s*/
      | int16_t xacc; /*< X acceleration (mg)*/
      | int16_t yacc; /*< Y acceleration (mg)*/
      | int16_t zacc; /*< Z acceleration (mg)*/
      | };
  TerrainZ : Inport
  <Ve> : Inport  Port=2
  <Xe> : Inport  Port=3
  <Eular(rad)> : Inport  Port=4
  <DCM> : Inport  Port=5
  <wb> : Inport  Port=6
  <dwb/dt> : Inport  Port=7
  <AccB> : Inport  Port=8
  <PosGPS> : Inport  Port=9
  <gravity> : Inport  Port=10
  <TempC> : Inport  Port=11
  <AirPressure> : Inport  Port=12
  <Rho> : Inport  Port=13
  <Windb> : Inport  Port=14
  MotorRads : Inport  Port=15
  <Fb> : Inport  Port=16
  PWM : Inport  Port=17
  Bus Creator : BusCreator  Inputs=11  OutDataTypeStr=Bus: MavVehileInfo
  Bus Selector8 : BusSelector  OutputSignals=lat,lon,alt  OutputAsBus=on
  Clock1 : Clock
  CopterID : Constant
  Data Type Conversion : DataTypeConversion  OutDataTypeStr=int32
  Data Type Conversion1 : DataTypeConversion  OutDataTypeStr=uint32
  Data Type Conversion{4..10} (7 alike) : DataTypeConversion  OutDataTypeStr=single
  Data Type Conversion11 : DataTypeConversion  OutDataTypeStr=double
  Data Type Conversion2 : DataTypeConversion  OutDataTypeStr=int32
  Data Type Conversion3 : DataTypeConversion  OutDataTypeStr=double
  Direction Cosine Matrix to Quaternions : sharedtransform/Direction Cosine Matrix  to Quaternions  aMode=aMode  action=None  tolerance=eps(2)
      settings: SourceProductBaseCode=AE
  Divide : Product  Inputs=*/
  Gain_clock : Gain  Gain=1E6
  HILGPSModel : Subsystem  Commented=on
  HILGPSModel1 : Subsystem
  HILSensorMavModel1 : Subsystem
  HILStateMavModel : Subsystem  Commented=on
  MagDec : Terminator
  MavHILStateQuat : Terminator  Commented=on
  ModelParam.uavMass : Constant  Value=ModelParam_uavMass
  Rate Transition : RateTransition  OutPortSampleTime=0.005
  SysTime : Terminator
  Terminator : Terminator
  UAVType : Constant  Value=ModelParam_uavType
  MavLinkSensorData : Outport  VectorParamsAs1DForOutWhenUnconnected=off
  Vehile3DInfo : Outport  Port=2  VectorParamsAs1DForOutWhenUnconnected=off
  HILGPSData : Outport  Port=3  VectorParamsAs1DForOutWhenUnconnected=off
  wires:
  <PosGPS>/1 -> HILStateMavModel/7(PosGPS), HILSensorMavModel1/5(GPSPos)
  <TempC>/1 -> HILSensorMavModel1/3(TempC)
  <AirPressure>/1 -> HILSensorMavModel1/4(pressure)
  Clock1/1 -> Data Type Conversion3/1, Gain_clock/1
  Data Type Conversion1/1 -> HILSensorMavModel1/1(time_usec), SysTime/1, HILGPSModel1/1(time_usec), HILGPSModel/1(time_usec), HILStateMavModel/1(time_usec)  "time_usec"
  <gravity>/1 -> HILSensorMavModel1/2(Gravity)
  <Rho>/1 -> HILSensorMavModel1/12(rho), HILStateMavModel/2(pho)
  Gain_clock/1 -> Data Type Conversion1/1
  <DCM>/1 -> HILSensorMavModel1/9(DCMbe), Direction Cosine Matrix to Quaternions/1
  <Eular(rad)>/1 -> HILGPSModel1/4(Euler), Data Type Conversion6/1
  <dwb/dt>/1 -> HILSensorMavModel1/7(dwt)
  <wb>/1 -> HILSensorMavModel1/6(wb), Data Type Conversion10/1, HILStateMavModel/6(wb)
  TerrainZ/1 -> Terminator/1
  CopterID/1 -> Data Type Conversion/1
  HILSensorMavModel1/2(MagDeclination) -> MagDec/1
  <AccB>/1 -> Data Type Conversion9/1
  Divide/1 -> HILSensorMavModel1/8(Ab)
  Data Type Conversion5/1 -> Bus Creator/5  "PosE"
  Data Type Conversion7/1 -> Bus Creator/7  "AngQuatern"
  Data Type Conversion4/1 -> Bus Creator/4  "VelE"
  Data Type Conversion9/1 -> Bus Creator/9  "AccB"
  Data Type Conversion10/1 -> Bus Creator/10  "RateB"
  PWM/1 -> HILSensorMavModel1/11(PWMin)
  Data Type Conversion11/1 -> Bus Creator/11  "PosGPS"
  Data Type Conversion6/1 -> Bus Creator/6  "AngEuler"
  Data Type Conversion/1 -> Bus Creator/1  "copterID"
  <Fb>/1 -> Divide/1
  MotorRads/1 -> Data Type Conversion8/1
  HILStateMavModel/1(stateOut) -> MavHILStateQuat/1
  Data Type Conversion8/1 -> Bus Creator/8  "MotorRPMS"
  Direction Cosine Matrix to Quaternions/1 -> Data Type Conversion7/1, HILStateMavModel/5(AngQuat)
  UAVType/1 -> Data Type Conversion2/1
  Data Type Conversion3/1 -> Bus Creator/3  "runnedTime"
  HILSensorMavModel1/3(acc) -> HILStateMavModel/8(Accb)
  ModelParam.uavMass/1 -> Divide/2
  Data Type Conversion2/1 -> Bus Creator/2  "vehicleType"
  HILSensorMavModel1/1(SensorOut) -> MavLinkSensorData/1
  <Windb>/1 -> HILSensorMavModel1/10(windB), HILStateMavModel/3(Vb)
  <Ve>/1 -> HILGPSModel1/2(Ve), HILGPSModel/2(Ve), HILStateMavModel/4(Ve), Data Type Conversion4/1
  <Xe>/1 -> HILGPSModel1/3(Xe), HILGPSModel/3(Xe), Data Type Conversion5/1
  Bus Creator/1 -> Rate Transition/1
  HILGPSModel1/1(HILGPSData) -> Bus Selector8/1, HILGPSData/1
  Rate Transition/1 -> Vehile3DInfo/1
  Bus Selector8/1 -> Data Type Conversion11/1

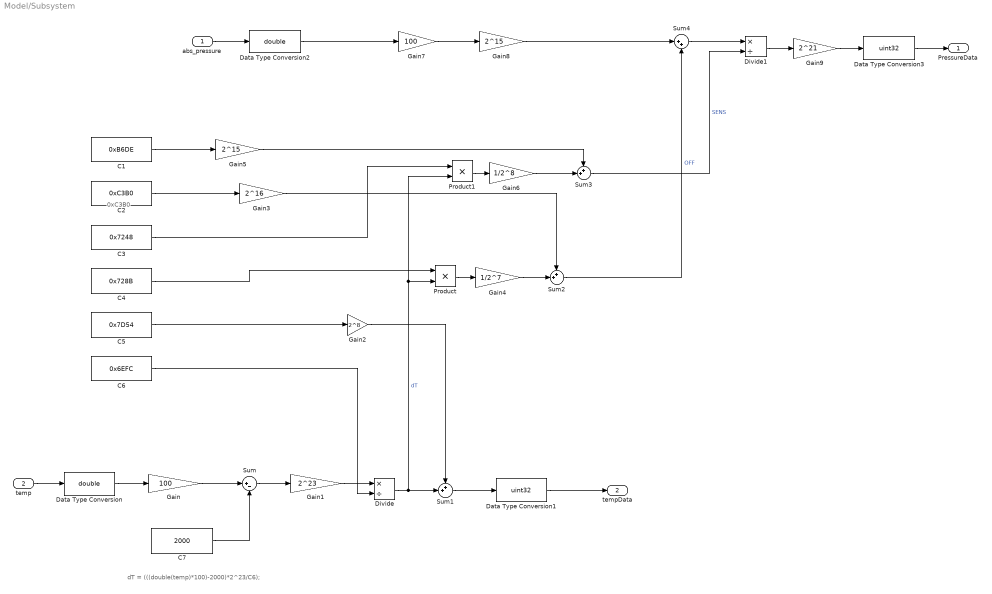
== system Model/Subsystem ==
  note: dT = (((double(temp)*100)-2000)*2^23/C6);
  note: 0xC3B0
  abs_pressure : Inport
  temp : Inport  Port=2
  C1 : Constant  Value=0xB6DE
  C2 : Constant  Value=0xC3B0
  C3 : Constant  Value=0x7248
  C4 : Constant  Value=0x728B
  C5 : Constant  Value=0x7D54
  C6 : Constant  Value=0x6EFC
  C7 : Constant  Value=2000
  Data Type Conversion : DataTypeConversion  OutDataTypeStr=double
  Data Type Conversion1 : DataTypeConversion  OutDataTypeStr=uint32
  Data Type Conversion2 : DataTypeConversion  OutDataTypeStr=double
  Data Type Conversion3 : DataTypeConversion  OutDataTypeStr=uint32
  Divide : Product  Inputs=*/
  Divide1 : Product  Inputs=*/
  Gain : Gain  Gain=100
  Gain1 : Gain  Gain=2^23
  Gain2 : Gain  Gain=2^8
  Gain3 : Gain  Gain=2^16
  Gain4 : Gain  Gain=1/2^7
  Gain5 : Gain  Gain=2^15
  Gain6 : Gain  Gain=1/2^8
  Gain7 : Gain  Gain=100
  Gain8 : Gain  Gain=2^15
  Gain9 : Gain  Gain=2^21
  Product : Product
  Product1 : Product
  Sum : Sum  Inputs=|+-
  Sum1 : Sum  Inputs=++|
  Sum2 : Sum  Inputs=++|
  Sum3 : Sum  Inputs=++|
  Sum4 : Sum  Inputs=|++
  PressureData : Outport
  tempData : Outport  Port=2
  wires:
  C6/1 -> Divide/2
  Divide/1 -> Product1/2, Product/2, Sum1/2  "dT"
  C2/1 -> Gain3/1
  Gain1/1 -> Divide/1
  Gain4/1 -> Sum2/2
  Gain6/1 -> Sum3/2
  C3/1 -> Product1/1
  C7/1 -> Sum/2
  Sum2/1 -> Sum4/2  "OFF"
  Gain8/1 -> Sum4/1
  Gain5/1 -> Sum3/1
  Sum/1 -> Gain1/1
  Sum1/1 -> Data Type Conversion1/1
  Gain7/1 -> Gain8/1
  Gain2/1 -> Sum1/1
  Divide1/1 -> Gain9/1
  Data Type Conversion1/1 -> tempData/1
  Product/1 -> Gain4/1
  Gain9/1 -> Data Type Conversion3/1
  C4/1 -> Product/1
  Product1/1 -> Gain6/1
  Data Type Conversion2/1 -> Gain7/1
  Sum4/1 -> Divide1/1
  Gain/1 -> Sum/1
  Gain3/1 -> Sum2/1
  C1/1 -> Gain5/1
  abs_pressure/1 -> Data Type Conversion2/1
  C5/1 -> Gain2/1
  Data Type Conversion/1 -> Gain/1
  temp/1 -> Data Type Conversion/1
  Sum3/1 -> Divide1/2  "SENS"
  Data Type Conversion3/1 -> PressureData/1

== system Model/6DOF/CaliModel ==
  step : Inport
  Accel_Mag : Inport  Port=2
  wb : Inport  Port=3
  DCM_be : Inport  Port=4
  Clock : Clock
  Demux : Demux  Outputs=3
  Direction Cosine Matrix to Quaternions : sharedtransform/Direction Cosine Matrix  to Quaternions  aMode=0  action=None  tolerance=eps(2)
      settings: SourceProductBaseCode=AE,PW,DR,MT,VE
  Ground Model : MATLAB Function  TreatAsAtomicUnit=on
  MATLAB Function : MATLAB Function  TreatAsAtomicUnit=on
  Mux : Mux  Inputs=3
  Quaternion Inverse : aerolibutil/Quaternion Inverse
  Quaternion Multiplication : aerolibutil/Quaternion Multiplication
  Reshape : Reshape
  Rotation Angles to Quaternions2 : sharedtransform/Rotation Angles to Quaternions  rotationOrder=ZYX  aMode=aMode
      settings: SourceProductBaseCode=AE,PW,DR,MT,VE
  Saturation : Saturate  UpperLimit=1  LowerLimit=-1
  Saturation1 : Saturate  UpperLimit=1  LowerLimit=-1
  Saturation2 : Saturate  UpperLimit=1  LowerLimit=-1
  Selector : Selector  InputPortWidth=3  IndexOptions=Index vector (dialog)  Indices=[3 2 1]  OutputSizes=1
  Fb : Outport
  Mb : Outport  Port=2
  wires:
  Direction Cosine Matrix to Quaternions/1 -> Quaternion Multiplication/2
  Clock/1 -> Ground Model/7(clock)
  step/1 -> Ground Model/6(step), MATLAB Function/1(step)
  Saturation/1 -> Mux/1
  Rotation Angles to Quaternions2/1 -> Quaternion Inverse/1
  Accel_Mag/1 -> MATLAB Function/2(Accel_Mag)
  Ground Model/1(F1) -> Fb/1
  Mux/1 -> Mb/1
  Quaternion Inverse/1 -> Quaternion Multiplication/1
  Demux/3 -> Saturation2/1
  Reshape/1 -> Ground Model/4(rotSpeed)
  Saturation1/1 -> Mux/2
  MATLAB Function/3(rotSpeed) -> Reshape/1
  Demux/2 -> Saturation1/1
  Quaternion Multiplication/1 -> Ground Model/2(Quet)
  MATLAB Function/4(rotTime) -> Ground Model/5(rotTime)
  Selector/1 -> Rotation Angles to Quaternions2/1
  MATLAB Function/1(desiredEuler) -> Selector/1
  Saturation2/1 -> Mux/3
  Ground Model/2(M1) -> Demux/1
  Demux/1 -> Saturation/1
  MATLAB Function/2(isRot) -> Ground Model/3(isRot)
  DCM_be/1 -> Direction Cosine Matrix to Quaternions/1
  wb/1 -> Ground Model/1(wb)

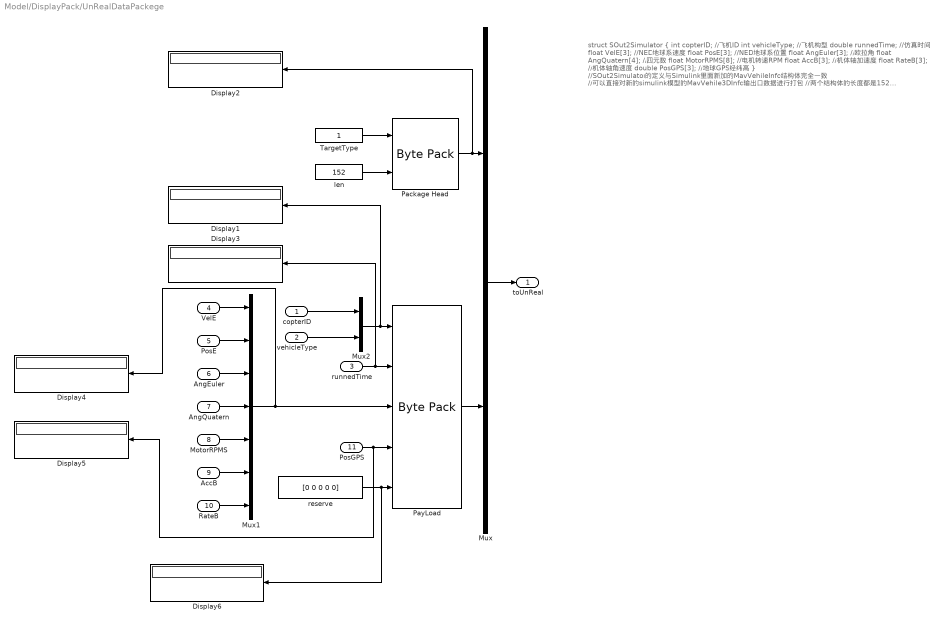
== system Model/DisplayPack/UnRealDataPackege ==
  note: struct SOut2Simulator
      | {
      | int copterID; //飞机ID
      | int vehicleType; //飞机构型
      | double runnedTime; //仿真时间
      | float VelE[3]; //NED地球系速度
      | float PosE[3]; //NED地球系位置
      | float AngEuler[3]; //欧拉角
      | float AngQuatern[4]; //四元数
      | float MotorRPMS[8]; //电机转速RPM
      | float AccB[3]; //机体轴加速度
      | float RateB[3]; //机体轴角速度
      | double PosGPS[3]; //地球GPS经纬高
      | }
      |
      | //SOut2Simulator的定义与Simulink里面新加的MavVehileInfo结构体完全一致
      | //可以直接对新的simulink模型的MavVehile3DInfo输出口数据进行打包
      | //两个结构体的长度都是152
      | sizeof(SOut2Simulator) = sizeof(MavVehileInfo) = 152
      |
      | 打包封装的结构体为
      | typedef struct _netDataShort
      | {
      | TargetType tg; //这里目前随便填，写1即可 uint32
      | int len; //这个长度为传输结构体长度，目前是152
      | char payload[192]; //这里面前152位存放了SOut2Simulator结构体数据，后面的40位保留
      | }netDataShort;
      |
      | //UDP包的总长度为200
      | sizeof(netDataShort) = 200
      |
      | //发送的UDP端口号为：20010
  copterID : Inport  PortDimensions=1
  vehicleType : Inport  Port=2  PortDimensions=1
  runnedTime : Inport  Port=3  PortDimensions=1
  "VelE " : Inport  Port=4  PortDimensions=3
  PosE : Inport  Port=5  PortDimensions=3
  AngEuler : Inport  Port=6  PortDimensions=3
  AngQuatern : Inport  Port=7  PortDimensions=4
  MotorRPMS : Inport  Port=8  PortDimensions=8
  AccB : Inport  Port=9  PortDimensions=3
  RateB : Inport  Port=10  PortDimensions=3
  PosGPS : Inport  Port=11  PortDimensions=3
  Display{1..6} (6 alike) : Display
  Mux : Mux  Inputs=2
  Mux1 : Mux  Inputs=7
  Mux2 : Mux  Inputs=2
  Package Head : etargetslib/Byte Pack  datatypes={'uint32','int32'}  byteAlign=4
  PayLoad : etargetslib/Byte Pack  datatypes={'int32','double','single','double','double'}  byteAlign=8
  TargetType : Constant  OutDataTypeStr=Inherit: Inherit via back propagation
  len : Constant  Value=152  OutDataTypeStr=Inherit: Inherit via back propagation
  reserve : Constant  Value=[0 0 0 0 0]  OutDataTypeStr=double  SampleTime=-1
  toUnReal : Outport
  wires:
  Package Head/1 -> Display2/1, Mux/1
  "VelE "/1 -> Mux1/1
  PosE/1 -> Mux1/2
  AngEuler/1 -> Mux1/3
  RateB/1 -> Mux1/7
  AccB/1 -> Mux1/6
  PayLoad/1 -> Mux/2
  Mux/1 -> toUnReal/1
  len/1 -> Package Head/2
  MotorRPMS/1 -> Mux1/5
  TargetType/1 -> Package Head/1
  AngQuatern/1 -> Mux1/4
  runnedTime/1 -> Display3/1, PayLoad/2
  PosGPS/1 -> PayLoad/4, Display5/1
  Mux1/1 -> Display4/1, PayLoad/3
  copterID/1 -> Mux2/1
  vehicleType/1 -> Mux2/2
  Mux2/1 -> Display1/1, PayLoad/1
  reserve/1 -> Display6/1, PayLoad/5

== system Model/Force and Moment Model/Body AeroCenter New ==
  wb : Inport
  Vb : Inport  Port=2
  Cd : Inport  Port=3
  CCm : Inport  Port=4
  uavDearo : Inport  Port=5
  Abs : Abs
  Abs1 : Abs
  Constant : Constant  Value=-1
  Constant1 : Constant  Value=0
  Demux : Demux  Outputs=3
  Gain : Gain  Gain=-1
  Mux : Mux  Inputs=3
  Product : Product  Inputs=****
  Product1 : Product  Inputs=****
  Product2 : Product
  Product3 : Product
  Sum : Sum  Inputs=|++
  Terminator : Terminator
  Fd : Outport  VectorParamsAs1DForOutWhenUnconnected=off
  Md : Outport  Port=2  VectorParamsAs1DForOutWhenUnconnected=off
  wires:
  Cd/1 -> Product/2
  wb/1 -> Abs1/1, Product1/3
  CCm/1 -> Product1/2
  Constant1/1 -> Mux/3
  uavDearo/1 -> Product3/2, Product2/2
  Product/1 -> Fd/1, Demux/1
  Abs1/1 -> Product1/4
  Demux/2 -> Product2/1
  Gain/1 -> Product3/1
  Vb/1 -> Abs/1, Product/3
  Abs/1 -> Product/4
  Product3/1 -> Mux/2
  Product1/1 -> Sum/1  "Md"
  Mux/1 -> Sum/2  "Mfd"
  Product2/1 -> Mux/1
  Demux/3 -> Terminator/1
  Sum/1 -> Md/1
  Constant/1 -> Product1/1, Product/1
  Demux/1 -> Gain/1

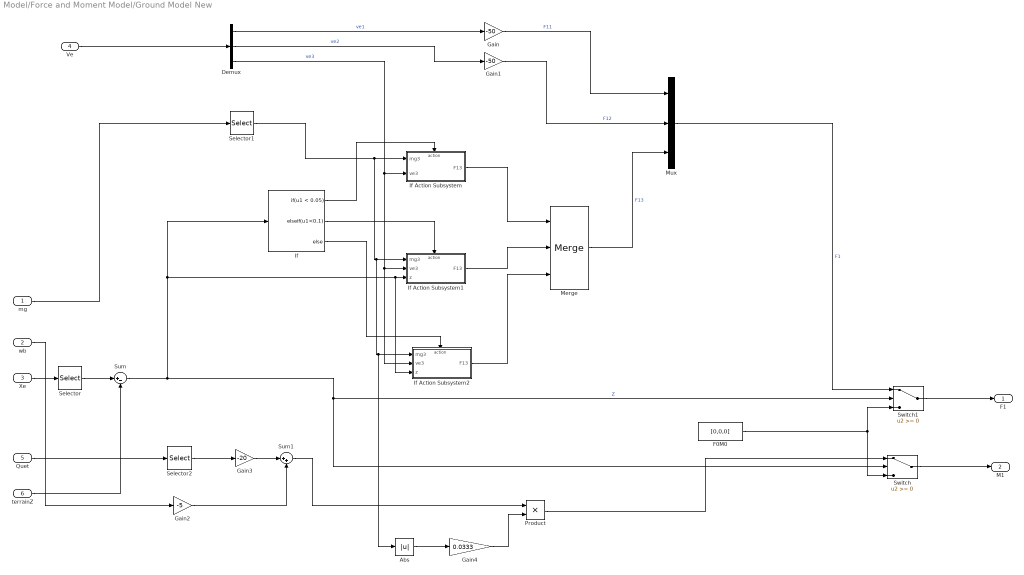
== system Model/Force and Moment Model/Ground Model New ==
  mg : Inport  PortDimensions=3
  wb : Inport  Port=2  PortDimensions=3
  Xe : Inport  Port=3  PortDimensions=3
  Ve : Inport  Port=4
  Quet : Inport  Port=5  PortDimensions=4
  terrainZ : Inport  Port=6
  Abs : Abs
  Demux : Demux  Outputs=3
  F0M0 : Constant  Value=[0,0,0]
  Gain : Gain  Gain=-50
  Gain1 : Gain  Gain=-50
  Gain2 : Gain  Gain=-5
  Gain3 : Gain  Gain=-20
  Gain4 : Gain  Gain=0.0333
  If : If  IfExpression=u1 < 0.05  ElseIfExpressions=u1<0.1
  If Action Subsystem : Subsystem  TreatAsAtomicUnit=on
  If Action Subsystem1 : Subsystem  TreatAsAtomicUnit=on
  If Action Subsystem2 : Subsystem  TreatAsAtomicUnit=on
  Merge : Merge  Inputs=3  InitialOutput=0
  Mux : Mux  Inputs=3
  Product : Product
  Selector : Selector  InputPortWidth=3  IndexOptions=Index vector (dialog)  Indices=[3]  OutputSizes=1
  Selector1 : Selector  InputPortWidth=3  IndexOptions=Index vector (dialog)  Indices=[3]  OutputSizes=1
  Selector2 : Selector  InputPortWidth=4  IndexOptions=Index vector (dialog)  Indices=[2:4]  OutputSizes=1
  Sum : Sum  Inputs=|+-
  Sum1 : Sum  Inputs=|++
  Switch : Switch
  Switch1 : Switch
  F1 : Outport  VectorParamsAs1DForOutWhenUnconnected=off
  M1 : Outport  Port=2  VectorParamsAs1DForOutWhenUnconnected=off
  wires:
  Gain2/1 -> Sum1/2
  Merge/1 -> Mux/3  "F13"
  Gain1/1 -> Mux/2  "F12"
  Switch1/1 -> F1/1
  Abs/1 -> Gain4/1
  Selector2/1 -> Gain3/1
  F0M0/1 -> Switch1/3, Switch/3
  Demux/1 -> Gain/1  "ve1"
  If Action Subsystem1/1(F13) -> Merge/2
  Quet/1 -> Selector2/1
  Ve/1 -> Demux/1
  Mux/1 -> Switch1/1  "F1"
  Gain3/1 -> Sum1/1
  Switch/1 -> M1/1
  Sum1/1 -> Product/1
  Gain4/1 -> Product/2
  Xe/1 -> Selector/1
  Demux/3 -> If Action Subsystem1/2(ve3), If Action Subsystem2/2(ve3), If Action Subsystem/2(ve3)  "ve3"
  Selector/1 -> Sum/1
  mg/1 -> Selector1/1
  wb/1 -> Gain2/1
  terrainZ/1 -> Sum/2
  Sum/1 -> Switch1/2, Switch/2, If Action Subsystem2/3(z), If Action Subsystem1/3(z), If/1  "Z"
  Product/1 -> Switch/1
  If/1 -> If Action Subsystem/Action
  If Action Subsystem2/1(F13) -> Merge/3
  If Action Subsystem/1(F13) -> Merge/1
  If/3 -> If Action Subsystem2/Action
  If/2 -> If Action Subsystem1/Action
  Gain/1 -> Mux/1  "F11"
  Selector1/1 -> If Action Subsystem/1(mg3), Abs/1, If Action Subsystem2/1(mg3), If Action Subsystem1/1(mg3)
  Demux/2 -> Gain1/1  "ve2"

== system Model/Force and Moment Model/Propeller Model Version New ==
  uavType : Inport
  MotorRads : Inport  Port=2
  R : Inport  Port=3
  Cm : Inport  Port=4
  Ct : Inport  Port=5
  Jm : Inport  Port=6
  wb : Inport  Port=7
  Constant1 : Constant
  Constant2 : Constant
  Display : Display
  Display1 : Display
  Display2 : Display
  Index Vector : MultiPortSwitch  DataPortOrder=Zero-based contiguous  Inputs=1  zeroidx=on
  Sum : Sum  Inputs=|+-
  TypeMotorAngMatrix : LookupNDDirect  InputsSelectThisObjectFromTable=Vector  Table=TypeMotorAngMatrix
  TypeMotorDirMatrix : LookupNDDirect  InputsSelectThisObjectFromTable=Vector  Table=TypeMotorDirMatrix
  TypeMotorNonVector : Constant  Value=TypeMotorNonVector
  While Iterator Subsystem : Subsystem  TreatAsAtomicUnit=on
  Fb : Outport  VectorParamsAs1DForOutWhenUnconnected=off
  Mb : Outport  Port=2  VectorParamsAs1DForOutWhenUnconnected=off
  wires:
  Constant1/1 -> While Iterator Subsystem/1(IC)
  Sum/1 -> TypeMotorAngMatrix/1, TypeMotorDirMatrix/1
  TypeMotorNonVector/1 -> Index Vector/2
  wb/1 -> While Iterator Subsystem/9(wb)
  TypeMotorDirMatrix/1 -> Display1/1, While Iterator Subsystem/3(TypeMotorDirVector)  "TypeMotorDirVector"
  MotorRads/1 -> While Iterator Subsystem/5(MotorRads)
  TypeMotorAngMatrix/1 -> Display2/1, While Iterator Subsystem/4(TypeMotorAngVector)  "TypeMotorAngVector"
  Jm/1 -> While Iterator Subsystem/10(Jm)
  Index Vector/1 -> Display/1, While Iterator Subsystem/2(Num)  "Num"
  Constant2/1 -> Sum/2
  Ct/1 -> While Iterator Subsystem/6(Ct)
  While Iterator Subsystem/2(Mb) -> Mb/1
  R/1 -> While Iterator Subsystem/8(R)
  Cm/1 -> While Iterator Subsystem/7(Cm)
  uavType/1 -> Sum/1, Index Vector/1
  While Iterator Subsystem/1(Fb) -> Fb/1

== system Model/Motor Model/MotorNonlinearDynamic1 ==
  Wb : Inport
  Cr : Inport  Port=2
  motorT : Inport  Port=3
  ModelInit_RPM : Inport  Port=4
  PWM : Inport  Port=5
  Minimum Throttle Cutoff : simulink/Logic and Bit Operations/Compare To Constant  relop=>=  const=ModelParam_motorMinThr  OutDataTypeStr=uint8
  Motor_Dynamics : Subsystem  TreatAsAtomicUnit=on
  Product : Product
  Product1 : Product
  Signal_Saturation : Saturate  UpperLimit=0.95  LowerLimit=0
  Sum1 : Sum  Inputs=++|
  radW : Outport  VectorParamsAs1DForOutWhenUnconnected=off
  wires:
  PWM/1 -> Signal_Saturation/1
  Motor_Dynamics/1(motor_rate_act) -> radW/1
  Product/1 -> Motor_Dynamics/1(motor_rate_d)
  Signal_Saturation/1 -> Product1/2, Minimum Throttle Cutoff/1
  Product1/1 -> Sum1/2
  Sum1/1 -> Product/1
  Wb/1 -> Sum1/1
  Minimum Throttle Cutoff/1 -> Product/2
  Cr/1 -> Product1/1
  motorT/1 -> Motor_Dynamics/3(motorT)
  ModelInit_RPM/1 -> Motor_Dynamics/2(ModelInit_RPM)
